simulink model "SkywalkerX8_Implementation"  (R2018a)
settings: Solver=FixedStepAuto  StartTime=0.0  StopTime=375  FixedStep=0.001  RelTol=1e-3
undefined symbols (not defined in the file): F, Light, MIL, SkywalkerX8
libraries: sensors x7, simulink_extras x3, aerolibwind2 x1
settings Model: Creator=David  LastModifiedBy=David

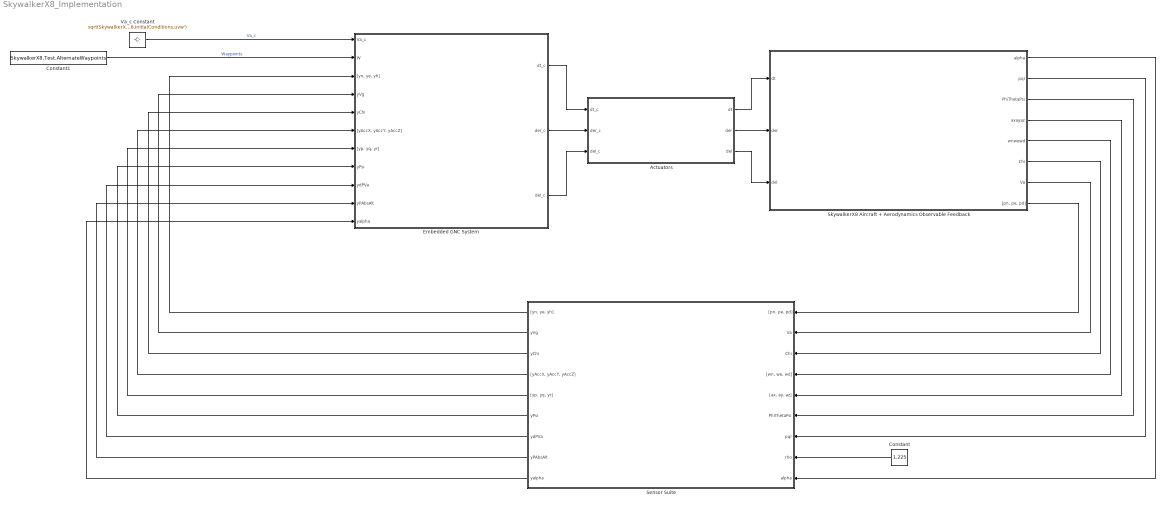
== system SkywalkerX8_Implementation ==
  Actuators : Subsystem
      mask Display:
      | image('actuators.jpg', 'center')
      | 
      | color('white')
      | 
      | port_label('input', 1, 'd_{t_c} (Unitless)', 'texmode', 'on')
      | port_label('input', 2, 'd_{{er}_c} (rad)', 'texmode', 'on')
      | port_label('input', 3, 'd_{{el}_c} (rad)', 'texmode', 'on')
      | 
      | port_label('output', 1, 'd_t (Unitless)', 'texmode', 'on')
      | port_label('output', 2, 'd_{er} (rad)', 'texmode', 'on')
      | port_label('output', 3, 'd_{el} (rad)', 'texmode', 'on')
  Constant : Constant  Value=1.225
  Constant1 : Constant  Value=SkywalkerX8.Test.AlternateWaypoints
  Embedded GNC System : Subsystem
      mask Display:
      | image('pixhawkv2-2.jpg')
      | 
      | color('cyan')
      | 
      | port_label('input', 1, 'Va_c (m/s)', 'texMode', 'On')
      | port_label('input', 2, '\bf{[W_i, W_{i+1} ..., W_N]} (m)', 'texMode', 'On')
      | port_label('input', 3, '[y_{GPS_N}, y_{GPS_E}, y_{GPS_h}] (m)', 'texMode', 'On')
      | port_label('input', 4, 'y_{GPS_{Vg}} (m/s)', 'texMode', 'On')
      | port_label('input', 5, 'y_{GPS_{\chi}} (rad)', 'texMode', 'On')
      | port_label('input', 6, '[y_{accel_x}, y_{accel_y}, y_{accel_z}] (m/s^2)', 'texMode', 'on')
      | port_label('input', 7, '[y_p, y_q, y_r] (rad/s)', 'texMode', 'on')
      | port_label('input', 8, 'y_{\psi} (rad)', 'texMode', 'on')
      | port_label('input', 9, 'y_{\DeltaP_{V_a}} (Pa)', 'texMode', 'on')
      | port_label('input', 10, 'y_{P_{abs}} (Pa)', 'texMode', 'on')
      | port_label('input', 11, 'y_\alpha (rad)', 'texMode', 'on')
      | 
      | port_label('output', 1, 'd_{t_c} (Unitless)', 'texmode', 'on')
      | port_label('output', 2, 'd_{{er}_c} (rad)', 'texmode', 'on')
      | port_label('output', 3, 'd_{{el}_c} (rad)', 'texmode', 'on')
  Sensor Suite : Subsystem
      mask Display:
      | image('telemetry.jpg')
      | 
      | color('cyan')
      | 
      | port_label('input', 1, '[p_N, p_E, p_D] (m)', 'texMode', 'On')
      | port_label('input', 2, 'V_a (m/s)', 'texMode', 'On')
      | port_label('input', 3, '\chi (rad)', 'texMode', 'On')
      | port_label('input', 4, '[w_N, w_E, w_D] (m/s)', 'texMode', 'On')
      | port_label('input', 5, '{\bfa_{inertial}} (m/s^2)', 'texMode', 'on')
      | port_label('input', 6, '[\phi, \theta, \psi] (rad)', 'texMode', 'on')
      | port_label('input', 7, '{\bf\omega_b} (rad/s)', 'texMode', 'on')
      | port_label('input', 8, '\rho (kg/m^3)', 'texMode', 'on')
      | port_label('input', 9, '\alpha (rad)', 'texMode', 'on')
      | 
      | port_label('output', 1, '[y_{GPS_N}, y_{GPS_E}, y_{GPS_h}] (m)', 'texMode', 'On')
      | port_label('output', 2, 'y_{GPS_{Vg}} (m/s)', 'texMode', 'On')
      | port_label('output', 3, 'y_{GPS_{\chi}} (rad)', 'texMode', 'On')
      | port_label('output', 4, '[y_{accel_x}, y_{accel_y}, y_{accel_z}] (m/s^2)', 'texMode', 'on')
      | port_label('output', 5, '[y_p, y_q, y_r] (rad/s)', 'texMode', 'on')
      | port_label('output', 6, 'y_{\psi} (rad)', 'texMode', 'on')
      | port_label('output', 7, 'y_{\DeltaP_{V_a}} (Pa)', 'texMode', 'on')
      | port_label('output', 8, 'y_{P_{abs}} (Pa)', 'texMode', 'on')
      | port_label('output', 9, 'y_\alpha (rad)', 'texMode', 'on')
  SkywalkerX8 Aircraft + Aerodynamics Observable Feedback : Subsystem
      mask Display:
      | image('x8SkySunset.png', 'center')
      | 
      | port_label('input', 1, '\delta_t (Unitless)', 'texmode', 'on')
      | port_label('input', 2, '\delta_e_r (rad)', 'texmode', 'on')
      | port_label('input', 3, '\delta_e_l (rad)', 'texmode', 'on')
      | 
      | port_label('output', 8, '[p_N, p_E, p_D] (m)', 'texMode', 'On')
      | port_label('output', 7, 'V_a (m/s)', 'texMode', 'On')
      | port_label('output', 6, '\chi (rad)', 'texMode', 'on')
      | port_label('output', 5, '[w_N, w_E, w_D] (m/s)', 'texMode', 'On')
      | port_label('output', 4, '{\bfa_{inertial}} (m/s^2)', 'texMode', 'on')
      | port_label('output', 3, '[\phi, \theta, \psi] (rad)', 'texMode', 'on')
      | port_label('output', 2, '{\bf\omega_b} (rad/s)', 'texMode', 'on')
      | port_label('output', 1, '\alpha (rad)', 'texMode', 'on')
  Va_c Constant : Constant  Value=sqrt(SkywalkerX8.InitialConditions.uvw*SkywalkerX8.InitialConditions.uvw')
  wires:
  SkywalkerX8 Aircraft + Aerodynamics Observable Feedback/3(PhiThetaPsi) -> Sensor Suite/6(PhiThetaPsi)
  SkywalkerX8 Aircraft + Aerodynamics Observable Feedback/8("[pn, pe, pd]") -> Sensor Suite/1("[pn, pe, pd]")
  SkywalkerX8 Aircraft + Aerodynamics Observable Feedback/6(Chi) -> Sensor Suite/3(Chi)
  SkywalkerX8 Aircraft + Aerodynamics Observable Feedback/2(pqr) -> Sensor Suite/7(pqr)
  Actuators/3(del) -> SkywalkerX8 Aircraft + Aerodynamics Observable Feedback/3(del)
  Constant/1 -> Sensor Suite/8(rho)
  SkywalkerX8 Aircraft + Aerodynamics Observable Feedback/4(axayaz) -> Sensor Suite/5("[ax, ay, az]")
  Actuators/1(dt) -> SkywalkerX8 Aircraft + Aerodynamics Observable Feedback/1(dt)
  SkywalkerX8 Aircraft + Aerodynamics Observable Feedback/5(wnwewd) -> Sensor Suite/4("[wn, we, wd]")
  SkywalkerX8 Aircraft + Aerodynamics Observable Feedback/7(Va) -> Sensor Suite/2(Va)
  SkywalkerX8 Aircraft + Aerodynamics Observable Feedback/1(alpha) -> Sensor Suite/9(alpha)
  Actuators/2(der) -> SkywalkerX8 Aircraft + Aerodynamics Observable Feedback/2(der)
  Va_c Constant/1 -> Embedded GNC System/1(Va_c)  "Va_c"
  Constant1/1 -> Embedded GNC System/2(W)  "Waypoints"
  Sensor Suite/1("[yn, ye, yh]") -> Embedded GNC System/3("[yn, ye, yh]")
  Sensor Suite/2(yVg) -> Embedded GNC System/4(yVg)
  Sensor Suite/3(yChi) -> Embedded GNC System/5(yChi)
  Sensor Suite/4("[yAccX, yAccY, yAccZ]") -> Embedded GNC System/6("[yAccX, yAccY, yAccZ]")
  Sensor Suite/5("[yp, yq, yr]") -> Embedded GNC System/7("[yp, yq, yr]")
  Sensor Suite/6(yPsi) -> Embedded GNC System/8(yPsi)
  Sensor Suite/7(ydPVa) -> Embedded GNC System/9(ydPVa)
  Sensor Suite/8(yPAbsAlt) -> Embedded GNC System/10(yPAbsAlt)
  Sensor Suite/9(yalpha) -> Embedded GNC System/11(yalpha)
  Embedded GNC System/1(dt_c) -> Actuators/1(dt_c)
  Embedded GNC System/2(der_c) -> Actuators/2(der_c)
  Embedded GNC System/3(del_c) -> Actuators/3(del_c)

== system SkywalkerX8_Implementation/Actuators ==
  dt_c : Inport
  der_c : Inport  Port=2
  del_c : Inport  Port=3
  Left Servo-Motor : Subsystem
      mask Display: image('servo.jpg', 'center')
  Motor Model : simulink_extras/Additional Linear/State-Space (with initial outputs)  A=SkywalkerX8.Actuators.Motor.SS.A  B=SkywalkerX8.Actuators.Motor.SS.B  C=SkywalkerX8.Actuators.Motor.SS.C  D=SkywalkerX8.Actuators.Motor.SS.D  U0=SkywalkerX8.InitialConditions.dt  Y0=SkywalkerX8.InitialConditions.dt  mask(State-Space with Initial Outputs){}
      settings: SourceProductName=Simulink  SourceProductBaseCode=SL
      mask Display: image('motor.jpg', 'center')
  Right Servo-Motor : Subsystem
      mask Display: image('servo.jpg', 'center')
  dt : Outport
  der : Outport  Port=2
  del : Outport  Port=3
  wires:
  del_c/1 -> Left Servo-Motor/1(del_c)
  Motor Model/1 -> dt/1
  Left Servo-Motor/1(del) -> del/1
  der_c/1 -> Right Servo-Motor/1(der_c)
  dt_c/1 -> Motor Model/1
  Right Servo-Motor/1(der) -> der/1

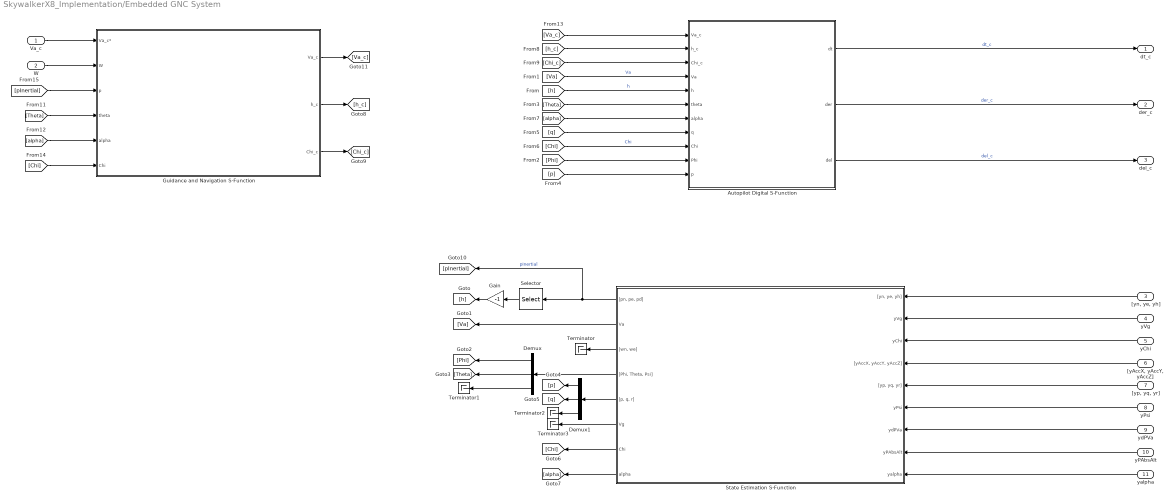
== system SkywalkerX8_Implementation/Embedded GNC System ==
  Va_c : Inport
  W : Inport  Port=2
  "[yn, ye, yh]" : Inport  Port=3
  yVg : Inport  Port=4
  yChi : Inport  Port=5
  "[yAccX, yAccY, yAccZ]" : Inport  Port=6
  "[yp, yq, yr]" : Inport  Port=7
  yPsi : Inport  Port=8
  ydPVa : Inport  Port=9
  yPAbsAlt : Inport  Port=10
  yalpha : Inport  Port=11
  Autopilot Digital S-Function : Subsystem
      mask help: Simulink:masks:GenSFuncDesc_MD
      mask Help: eval('feval(''rtwprivate'',''rtwhelpview'',''rtw_sfcn_block'')');
      mask Display:
      | image('autopilot.png', 'center')
      | 
      | port_label('output', 1, '\delta_t (Unitless)', 'texmode', 'on')
      | port_label('output', 2, '\delta_e_r (rad)', 'texmode', 'on')
      | port_label('output', 3, '\delta_e_l (rad)', 'texmode', 'on')
      | 
      | port_label('input', 1, 'V_{a_c} (m/s)', 'texmode', 'on')
      | port_label('input', 2, 'h_c (m)', 'texmode', 'on')
      | port_label('input', 3, '\chi_c (rad)', 'texmode', 'on')
      | port_label('input', 4, 'V_a (m/s)', 'texmode', 'on')
      | port_label('input', 5, 'Altitude (m)', 'texmode', 'on')
      | port_label('input', 6, '\theta (rad)', 'texmode', 'on')
      | port_label('input', 7, '\alpha (rad)', 'texmode', 'on')
      | port_label('input', 8, 'q (rad/s)', 'texmode', 'on')
      | port_label('input', 9, '\chi (rad)', 'texmode', 'on')
      | port_label('input', 10, '\phi (rad)', 'texmode', 'on')
      | port_label('input', 11, 'p (rad/s)', 'texmode', 'on')
  Demux : Demux  Outputs=3
  Demux1 : Demux  Outputs=3
  Gain : Gain  Gain=-1
  Guidance and Navigation S-Function : Subsystem
      mask help: Simulink:masks:GenSFuncDesc_MD
      mask Help: eval('feval(''rtwprivate'',''rtwhelpview'',''rtw_sfcn_block'')');
      mask Display:
      | image('Aircraft-navigation.jpg')
      | 
      | color('green')
      | 
      | port_label('input', 1, 'Va_c', 'texMode', 'On')
      | port_label('input', 2, '\bf{[W_1, W_2, ... W_n]}', 'texMode', 'On')
      | port_label('input', 3, '\bf{p}', 'texMode', 'On')
      | port_label('input', 4, '\theta', 'texMode', 'On')
      | port_label('input', 5, '\alpha', 'texMode', 'On')
      | port_label('input', 6, '\chi', 'texMode', 'On')
      | 
      | port_label('output', 1, 'Va_c', 'texMode', 'On')
      | port_label('output', 2, 'h_c', 'texMode', 'On')
      | port_label('output', 3, '\chi_c', 'texMode', 'On')
  Selector : Selector  InputPortWidth=3  IndexOptions=Index vector (dialog)  Indices=3  OutputSizes=1
  State Estimation S-Function : Subsystem
      mask help: Simulink:masks:GenSFuncDesc_MD
      mask Help: eval('feval(''rtwprivate'',''rtwhelpview'',''rtw_sfcn_block'')');
      mask Display:
      | image('state_estimate.jpg', 'center')
      | 
      | port_label('input', 1, '[y_{GPS_N}, y_{GPS_E}, y_{GPS_h}] (m)', 'texMode', 'On')
      | port_label('input', 2, 'y_{GPS_{Vg}} (m/s)', 'texMode', 'On')
      | port_label('input', 3, 'y_{GPS_{\chi}} (rad)', 'texMode', 'On')
      | port_label('input', 4, '[y_{accel_x}, y_{accel_y}, y_{accel_z}] (m/s^2)', 'texMode', 'on')
      | port_label('input', 5, '[y_p, y_q, y_r] (rad/s)', 'texMode', 'on')
      | port_label('input', 6, 'y_{\psi} (rad)', 'texMode', 'on')
      | port_label('input', 7, 'y_{\DeltaP_{V_a}} (Pa)', 'texMode', 'on')
      | port_label('input', 8, 'y_{P_{abs}} (Pa)', 'texMode', 'on')
      | port_label('input', 9, 'y_{\alpha} (rad)', 'texMode', 'on')
      | 
      | port_label('output', 1, '[p_N, p_E, p_D] (m)', 'texMode', 'On')
      | port_label('output', 2, 'V_a (m/s)', 'texMode', 'On')
      | port_label('output', 3, '[w_N, w_E] (m/s)', 'texMode', 'On')
      | port_label('output', 4, '[\phi, \theta, \psi] (rad)', 'texMode', 'on')
      | port_label('output', 5, '{\bf\omega_b} (rad/s)', 'texMode', 'on')
      | port_label('output', 6, 'V_g (m/s)', 'texMode', 'on')
      | port_label('output', 7, '\chi (rad)', 'texMode', 'on')
      | port_label('output', 8, '\alpha (rad)', 'texMode', 'on')
  Terminator{,1..3} (4 alike) : Terminator
  dt_c : Outport
  der_c : Outport  Port=2
  del_c : Outport  Port=3
  wires:
  [pInertial] -> Guidance and Navigation S-Function/3(p)
  "[yAccX, yAccY, yAccZ]"/1 -> State Estimation S-Function/4("[yAccX, yAccY, yAccZ]")
  State Estimation S-Function/6(Vg) -> Terminator3/1
  State Estimation S-Function/1("[pn, pe, pd]") -> [pInertial], Selector/1  "pInertial"
  [alpha] -> Autopilot Digital S-Function/7(alpha)
  Demux/2 -> [Theta]
  Demux1/3 -> Terminator2/1
  [h_c] -> Autopilot Digital S-Function/2(h_c)
  Demux/1 -> [Phi]
  Demux1/1 -> [p]
  [Chi] -> Guidance and Navigation S-Function/6(Chi)
  [q] -> Autopilot Digital S-Function/8(q)
  Demux/3 -> Terminator1/1
  [Phi] -> Autopilot Digital S-Function/10(Phi)
  yVg/1 -> State Estimation S-Function/2(yVg)
  W/1 -> Guidance and Navigation S-Function/2(W)
  Gain/1 -> [h]
  yPAbsAlt/1 -> State Estimation S-Function/8(yPAbsAlt)
  Selector/1 -> Gain/1
  Demux1/2 -> [q]
  [Chi_c] -> Autopilot Digital S-Function/3(Chi_c)
  "[yp, yq, yr]"/1 -> State Estimation S-Function/5("[yp, yq, yr]")
  yChi/1 -> State Estimation S-Function/3(yChi)
  [alpha] -> Guidance and Navigation S-Function/5(alpha)
  Guidance and Navigation S-Function/1(Va_c) -> [Va_c]
  Guidance and Navigation S-Function/3(Chi_c) -> [Chi_c]
  State Estimation S-Function/2(Va) -> [Va]
  State Estimation S-Function/7(Chi) -> [Chi]
  [Theta] -> Guidance and Navigation S-Function/4(theta)
  Guidance and Navigation S-Function/2(h_c) -> [h_c]
  State Estimation S-Function/4("[Phi, Theta, Psi]") -> Demux/1
  Autopilot Digital S-Function/1(dt) -> dt_c/1  "dt_c"
  State Estimation S-Function/3("[wn, we]") -> Terminator/1
  Autopilot Digital S-Function/2(der) -> der_c/1  "der_c"
  State Estimation S-Function/8(alpha) -> [alpha]
  Va_c/1 -> Guidance and Navigation S-Function/1(Va_c*)
  Autopilot Digital S-Function/3(del) -> del_c/1  "del_c"
  State Estimation S-Function/5("[p, q, r]") -> Demux1/1
  "[yn, ye, yh]"/1 -> State Estimation S-Function/1("[yn, ye, yh]")
  [Theta] -> Autopilot Digital S-Function/6(theta)
  [Va_c] -> Autopilot Digital S-Function/1(Va_c)
  yPsi/1 -> State Estimation S-Function/6(yPsi)
  [Va] -> Autopilot Digital S-Function/4(Va)  "Va"
  [p] -> Autopilot Digital S-Function/11(p)
  [h] -> Autopilot Digital S-Function/5(h)  "h"
  [Chi] -> Autopilot Digital S-Function/9(Chi)  "Chi"
  yalpha/1 -> State Estimation S-Function/9(yalpha)
  ydPVa/1 -> State Estimation S-Function/7(ydPVa)

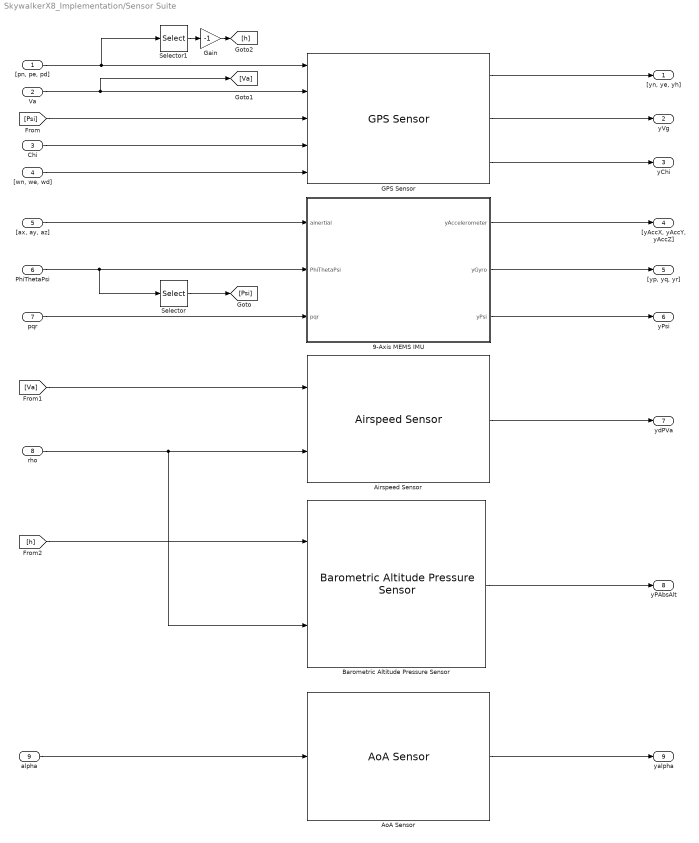
== system SkywalkerX8_Implementation/Sensor Suite ==
  "[pn, pe, pd]" : Inport
  Va : Inport  Port=2
  Chi : Inport  Port=3
  "[wn, we, wd]" : Inport  Port=4
  "[ax, ay, az]" : Inport  Port=5
  PhiThetaPsi : Inport  Port=6
  pqr : Inport  Port=7
  rho : Inport  Port=8
  alpha : Inport  Port=9
  9-Axis MEMS IMU : Subsystem
      mask Display:
      | image('VNAV_IMU.jpg')
      | 
      | color('green')
      | 
      | port_label('input', 1, '{\bfa_{inertial}} (m/s^2)', 'texMode', 'on')
      | port_label('input', 2, '[\phi, \theta, \psi] (rad)', 'texMode', 'on')
      | port_label('input', 3, '{\bf\omega_b} (rad/s)', 'texMode', 'on')
      | 
      | port_label('output', 1, '[y_{accel_x}, y_{accel_y}, y_{accel_z}] (m/s^2)', 'texMode', 'on')
      | port_label('output', 2, '[y_p, y_q, y_r] (rad/s)', 'texMode', 'on')
      | port_label('output', 3, 'y_{\psi} (rad)', 'texMode', 'on')
  Airspeed Sensor : sensors/Airspeed Sensor  SampleTime=SkywalkerX8.Sensors.AirspeedPressure.SampleTime  diffPressureStdDev=SkywalkerX8.Sensors.AirspeedPressure.StdDev  diffPressureBandwidthHz=SkywalkerX8.Sensors.AirspeedPressure.BandwidthHz  diffPressureInit=SkywalkerX8.Sensors.AirspeedPressure.InitialCondition  diffPressureUpperSaturation=SkywalkerX8.Sensors.AirspeedPressure.UpperSat  diffPressureLowerSaturation=SkywalkerX8.Sensors.AirspeedPressure.LowerSat  diffPressureResolution=SkywalkerX8.Sensors.AirspeedPressure.Resolution
  AoA Sensor : sensors/AoA Sensor  SampleTime=SkywalkerX8.Sensors.AoA.SampleTime  alphaStdDev=SkywalkerX8.Sensors.AoA.StdDev  alphaBandwidthHz=SkywalkerX8.Sensors.AoA.BandwidthHz  alphaInit=SkywalkerX8.Sensors.AoA.InitialCondition  alphaUpperSaturation=SkywalkerX8.Sensors.AoA.UpperSat  alphaLowerSaturation=SkywalkerX8.Sensors.AoA.LowerSat  alphaResolution=SkywalkerX8.Sensors.AoA.Resolution
  Barometric Altitude Pressure Sensor : sensors/Barometric Altitude Pressure Sensor  g=SkywalkerX8.System.Gravity  SampleTime=SkywalkerX8.Sensors.AltitudePressure.SampleTime  absPressureStdDev=SkywalkerX8.Sensors.AltitudePressure.StdDev  absPressureBandwidthHz=SkywalkerX8.Sensors.AltitudePressure.BandwidthHz  absPressureInit=SkywalkerX8.Sensors.AltitudePressure.InitialCondition  absPressureUpperSaturation=SkywalkerX8.Sensors.AltitudePressure.UpperSat  absPressureLowerSaturation=SkywalkerX8.Sensors.AltitudePressure.LowerSat  absPressureResolution=SkywalkerX8.Sensors.AltitudePressure.Resolution
  GPS Sensor : sensors/GPS Sensor  SampleTime=SkywalkerX8.Sensors.GPS.SampleTime  pnInit=SkywalkerX8.Sensors.GPS.pnInit  peInit=SkywalkerX8.Sensors.GPS.peInit  pdInit=SkywalkerX8.Sensors.GPS.pdInit  VgInit=SkywalkerX8.Sensors.GPS.VgInit  ChiInit=SkywalkerX8.Sensors.GPS.ChiInit  GPSNStdDev=SkywalkerX8.Sensors.GPS.North.StdDev  OneOverkGPSN=SkywalkerX8.Sensors.GPS.North.TimeConstant  GPSEStdDev=SkywalkerX8.Sensors.GPS.East.StdDev  OneOverkGPSE=SkywalkerX8.Sensors.GPS.East.TimeConstant  GPSAltStdDev=SkywalkerX8.Sensors.GPS.Alt.StdDev  OneOverkGPSAlt=SkywalkerX8.Sensors.GPS.Alt.TimeConstant  GPSVStdDev=SkywalkerX8.Sensors.GPS.Velocity.StdDev
  Gain : Gain  Gain=-1
  Selector : Selector  InputPortWidth=3  IndexOptions=Index vector (dialog)  Indices=3  OutputSizes=1
  Selector1 : Selector  InputPortWidth=3  IndexOptions=Index vector (dialog)  Indices=3  OutputSizes=1
  "[yn, ye, yh]" : Outport
  yVg : Outport  Port=2
  yChi : Outport  Port=3
  "[yAccX, yAccY, yAccZ]" : Outport  Port=4
  "[yp, yq, yr]" : Outport  Port=5
  yPsi : Outport  Port=6
  ydPVa : Outport  Port=7
  yPAbsAlt : Outport  Port=8
  yalpha : Outport  Port=9
  wires:
  "[pn, pe, pd]"/1 -> GPS Sensor/1, Selector1/1
  Va/1 -> [Va], GPS Sensor/2
  PhiThetaPsi/1 -> 9-Axis MEMS IMU/2(PhiThetaPsi), Selector/1
  Airspeed Sensor/1 -> ydPVa/1
  [Psi] -> GPS Sensor/3
  Selector1/1 -> Gain/1
  rho/1 -> Barometric Altitude Pressure Sensor/2, Airspeed Sensor/2
  GPS Sensor/3 -> yChi/1
  Selector/1 -> [Psi]
  [h] -> Barometric Altitude Pressure Sensor/1
  9-Axis MEMS IMU/3(yPsi) -> yPsi/1
  [Va] -> Airspeed Sensor/1
  pqr/1 -> 9-Axis MEMS IMU/3(pqr)
  9-Axis MEMS IMU/2(yGyro) -> "[yp, yq, yr]"/1
  "[wn, we, wd]"/1 -> GPS Sensor/5
  Barometric Altitude Pressure Sensor/1 -> yPAbsAlt/1
  GPS Sensor/1 -> "[yn, ye, yh]"/1
  Gain/1 -> [h]
  GPS Sensor/2 -> yVg/1
  "[ax, ay, az]"/1 -> 9-Axis MEMS IMU/1(ainertial)
  9-Axis MEMS IMU/1(yAccelerometer) -> "[yAccX, yAccY, yAccZ]"/1
  AoA Sensor/1 -> yalpha/1
  alpha/1 -> AoA Sensor/1
  Chi/1 -> GPS Sensor/4

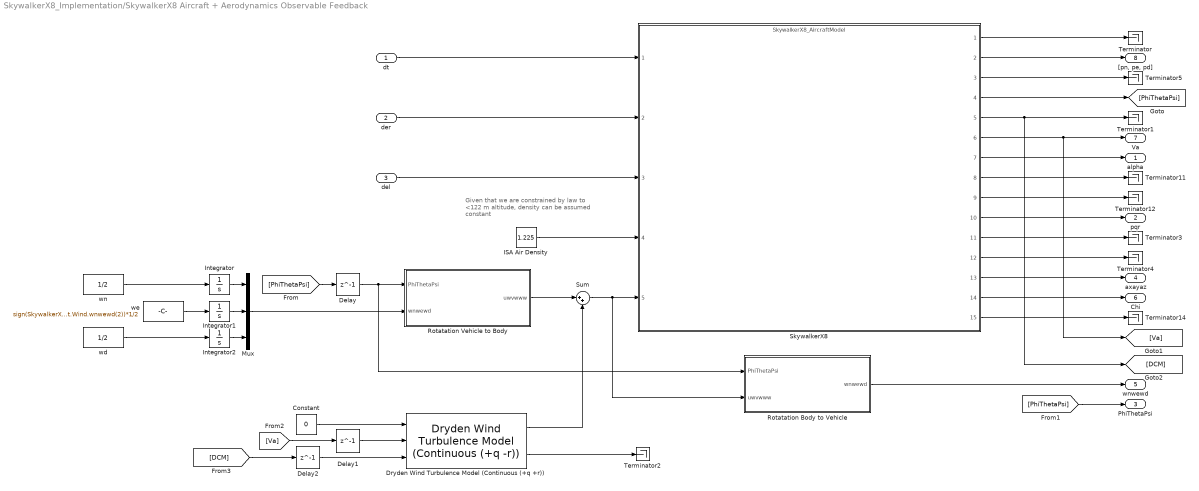
== system SkywalkerX8_Implementation/SkywalkerX8 Aircraft + Aerodynamics Observable Feedback ==
  note: Given that we are constrained by law to
      | <122 m altitude, density can be assumed
      | constant
  dt : Inport
  der : Inport  Port=2
  del : Inport  Port=3
  Constant : Constant  Value=0
  Delay : Delay  DelayLength=1  InitialCondition=SkywalkerX8.InitialConditions.PhiThetaPsi
  Delay1 : Delay  DelayLength=1  InitialCondition=sqrt(SkywalkerX8.InitialConditions.uvw*SkywalkerX8.InitialConditions.uvw')
  Delay2 : Delay  DelayLength=1  InitialCondition=zeros(3, 3)
  Dryden Wind Turbulence Model (Continuous (+q +r)) : aerolibwind2/Dryden Wind Turbulence Model  (Continuous (+q -r))  units=Metric (MKS)  spec=MIL-F-8785C  model=Continuous Dryden (+q +r)  W20=sqrt(SkywalkerX8.Ambient.Wind.wnwewd*SkywalkerX8.Ambient.Wind.wnwewd')  Wdeg=rad2deg(atan2(SkywalkerX8.Ambient.Wind.wnwewd(2), SkywalkerX8.Ambient.Wind.wnwewd(1)))  TurbProb=10^-2 - Light  L_high=533.4  Wingspan=SkywalkerX8.Geometry.b  ts=0.001  Seed=[23341 23342 23343 23344]  T_on=on
      settings: SourceProductName=Aerospace Blockset
  ISA Air Density : Constant  Value=1.225
  Integrator : Integrator  LimitOutput=on  UpperSaturationLimit=(SkywalkerX8.Ambient.Wind.wnwewd(1)>0)*SkywalkerX8.Ambient.Wind.wnwewd(1)+1E-06  LowerSaturationLimit=(SkywalkerX8.Ambient.Wind.wnwewd(1)<0)*SkywalkerX8.Ambient.Wind.wnwewd(1)-1E-06
  Integrator1 : Integrator  LimitOutput=on  UpperSaturationLimit=(SkywalkerX8.Ambient.Wind.wnwewd(2)>0)*SkywalkerX8.Ambient.Wind.wnwewd(2)+1E-06  LowerSaturationLimit=(SkywalkerX8.Ambient.Wind.wnwewd(2)<0)*SkywalkerX8.Ambient.Wind.wnwewd(2)-1E-06
  Integrator2 : Integrator  LimitOutput=on  UpperSaturationLimit=(SkywalkerX8.Ambient.Wind.wnwewd(3)>0)*SkywalkerX8.Ambient.Wind.wnwewd(3)+1E-06  LowerSaturationLimit=(SkywalkerX8.Ambient.Wind.wnwewd(3)<0)*SkywalkerX8.Ambient.Wind.wnwewd(3)-1E-06
  Mux : Mux  Inputs=3
  Rotatation Body to Vehicle : MATLAB Function  TreatAsAtomicUnit=on
  Rotatation Vehicle to Body : MATLAB Function  TreatAsAtomicUnit=on
  SkywalkerX8 : ModelReference  ModelNameDialog=SkywalkerX8_AircraftModel  ModelReferenceVersion=1.367
      mask Display:
      | image('C:\MATLAB\masters\icons\Skywalker Main Block Icon.png', 'center')
      | 
      | color('cyan')
      | 
      | port_label('input', 1, 'k_{motor} (Unitless)', 'texmode', 'on')
      | port_label('input', 2, '\delta_{er} (rad)', 'texmode', 'on')
      | port_label('input', 3, '\delta_{el} (rad)', 'texmode', 'on')
      | port_label('input', 4, '\rho (kg/m^3)', 'texmode', 'on')
      | port_label('input', 5, '{\bf V_w^b} (m/s)', 'texmode', 'on')
      | 
      | port_label('output', 1, '{\bf V_e} (m/s)', 'texmode', 'on')
      | port_label('output', 2, '{\bf X_e} (m)', 'texmode', 'on')
      | port_label('output', 3, 'Altitude (m)', 'texmode', 'on')
      | port_label('output', 4, '\phi \theta \psi (rad)', 'texmode', 'on')
      | port_label('output', 5, 'R_{inertial}^{body}', 'texmode', 'on')
      | port_label('output', 6, 'V_a (m/s)', 'texmode', 'on')
      | port_label('output', 7, 'alpha (rad)', 'texmode', 'on')
      | port_label('output', 8, 'beta (rad)', 'texmode', 'on')
      | port_label('output', 9, '{\bf V_b} (m/s)', 'texmode', 'on')
      | port_label('output', 10, '{\bf \omega_b} (rad/s)', 'texmode', 'on')
      | port_label('output', 11, '{\bf \delta\omega_b/\deltat} (rad/s^2)', 'texmode', 'on')
      | port_label('output', 12, '{\bf a_{body}} (m/s^2)', 'texmode', 'on')
      | port_label('output', 13, '{\bf a_{inertial}} (m/s^2)', 'texmode', 'on')
      | port_label('output', 14, '\chi (rad)', 'texmode', 'on')
      | port_label('output', 15, '\chi_c (rad)', 'texmode', 'on')
  Sum : Sum  Inputs=|++
  Terminator{,1..5,11..12,14} (9 alike) : Terminator
  wd : Constant  Value=1/2
  we : Constant  Value=sign(SkywalkerX8.Ambient.Wind.wnwewd(2))*1/2
  wn : Constant  Value=1/2
  alpha : Outport
  pqr : Outport  Port=2
  PhiThetaPsi : Outport  Port=3
  axayaz : Outport  Port=4
  wnwewd : Outport  Port=5
  Chi : Outport  Port=6
  Va : Outport  Port=7
  "[pn, pe, pd]" : Outport  Port=8
  wires:
  SkywalkerX8/12 -> Terminator4/1
  SkywalkerX8/13 -> axayaz/1
  Rotatation Vehicle to Body/1(uwvwww) -> Sum/1
  SkywalkerX8/11 -> Terminator3/1
  SkywalkerX8/6 -> [Va], Va/1
  SkywalkerX8/1 -> Terminator/1
  SkywalkerX8/5 -> [DCM], Terminator1/1
  SkywalkerX8/7 -> alpha/1
  dt/1 -> SkywalkerX8/1
  SkywalkerX8/8 -> Terminator11/1
  SkywalkerX8/3 -> Terminator5/1
  SkywalkerX8/9 -> Terminator12/1
  SkywalkerX8/2 -> "[pn, pe, pd]"/1
  SkywalkerX8/4 -> [PhiThetaPsi]
  SkywalkerX8/15 -> Terminator14/1
  SkywalkerX8/10 -> pqr/1
  ISA Air Density/1 -> SkywalkerX8/4
  SkywalkerX8/14 -> Chi/1
  del/1 -> SkywalkerX8/3
  der/1 -> SkywalkerX8/2
  Mux/1 -> Rotatation Vehicle to Body/2(wnwewd)
  [PhiThetaPsi] -> Delay/1
  [PhiThetaPsi] -> PhiThetaPsi/1
  Delay/1 -> Rotatation Body to Vehicle/1(PhiThetaPsi), Rotatation Vehicle to Body/1(PhiThetaPsi)
  Constant/1 -> Dryden Wind Turbulence Model (Continuous (+q +r))/1
  [Va] -> Delay1/1
  [DCM] -> Delay2/1
  Dryden Wind Turbulence Model (Continuous (+q +r))/2 -> Terminator2/1
  Sum/1 -> Rotatation Body to Vehicle/2(uwvwww), SkywalkerX8/5
  Dryden Wind Turbulence Model (Continuous (+q +r))/1 -> Sum/2
  Delay1/1 -> Dryden Wind Turbulence Model (Continuous (+q +r))/2
  Delay2/1 -> Dryden Wind Turbulence Model (Continuous (+q +r))/3
  Rotatation Body to Vehicle/1(wnwewd) -> wnwewd/1
  wd/1 -> Integrator2/1
  Integrator2/1 -> Mux/3
  wn/1 -> Integrator/1
  Integrator/1 -> Mux/1
  we/1 -> Integrator1/1
  Integrator1/1 -> Mux/2

== system SkywalkerX8_Implementation/Actuators/Left Servo-Motor ==
  del_c : Inport
  Rate Limiter : RateLimiter  Commented=through  RisingSlewLimit=SkywalkerX8.Actuators.Servos.RateLimit  FallingSlewLimit=-SkywalkerX8.Actuators.Servos.RateLimit  SampleTimeMode=inherited  InitialCondition=SkywalkerX8.InitialConditions.de*0.5 + SkywalkerX8.InitialConditions.da*0.5
  Saturation : Saturate  UpperLimit=SkywalkerX8.Actuators.Servos.UpperSaturation  LowerLimit=SkywalkerX8.Actuators.Servos.LowerSaturation
  Second Order Servo-Motor Model : simulink_extras/Additional Linear/State-Space (with initial outputs)  A=SkywalkerX8.Actuators.Servos.SS.A  B=SkywalkerX8.Actuators.Servos.SS.B  C=SkywalkerX8.Actuators.Servos.SS.C  D=SkywalkerX8.Actuators.Servos.SS.D  U0=(SkywalkerX8.InitialConditions.de*0.5 + SkywalkerX8.InitialConditions.da*0.5)  Y0=(SkywalkerX8.InitialConditions.de*0.5 + SkywalkerX8.InitialConditions.da*0.5)
      settings: SourceProductName=Simulink  SourceProductBaseCode=SL
  del : Outport
  wires:
  Rate Limiter/1 -> Saturation/1
  del_c/1 -> Second Order Servo-Motor Model/1
  Saturation/1 -> del/1
  Second Order Servo-Motor Model/1 -> Rate Limiter/1

== system SkywalkerX8_Implementation/Actuators/Right Servo-Motor ==
  der_c : Inport
  Rate Limiter : RateLimiter  Commented=through  RisingSlewLimit=SkywalkerX8.Actuators.Servos.RateLimit  FallingSlewLimit=-SkywalkerX8.Actuators.Servos.RateLimit  SampleTimeMode=inherited  InitialCondition=SkywalkerX8.InitialConditions.de*0.5 - SkywalkerX8.InitialConditions.da*0.5
  Saturation : Saturate  UpperLimit=SkywalkerX8.Actuators.Servos.UpperSaturation  LowerLimit=SkywalkerX8.Actuators.Servos.LowerSaturation
  Second Order Servo-Motor Model : simulink_extras/Additional Linear/State-Space (with initial outputs)  A=SkywalkerX8.Actuators.Servos.SS.A  B=SkywalkerX8.Actuators.Servos.SS.B  C=SkywalkerX8.Actuators.Servos.SS.C  D=SkywalkerX8.Actuators.Servos.SS.D  U0=(SkywalkerX8.InitialConditions.de*0.5 - SkywalkerX8.InitialConditions.da*0.5)  Y0=(SkywalkerX8.InitialConditions.de*0.5 - SkywalkerX8.InitialConditions.da*0.5)
      settings: SourceProductName=Simulink  SourceProductBaseCode=SL
  der : Outport
  wires:
  Rate Limiter/1 -> Saturation/1
  der_c/1 -> Second Order Servo-Motor Model/1
  Second Order Servo-Motor Model/1 -> Rate Limiter/1
  Saturation/1 -> der/1

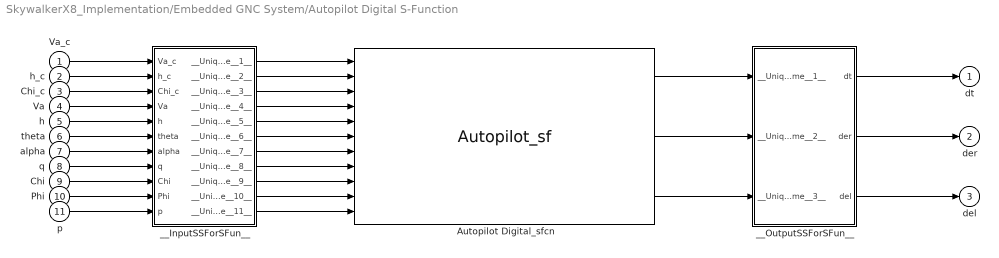
== system SkywalkerX8_Implementation/Embedded GNC System/Autopilot Digital S-Function ==
  Va_c : Inport
  h_c : Inport  Port=2
  Chi_c : Inport  Port=3
  Va : Inport  Port=4
  h : Inport  Port=5
  theta : Inport  Port=6
  alpha : Inport  Port=7
  q : Inport  Port=8
  Chi : Inport  Port=9
  Phi : Inport  Port=10
  p : Inport  Port=11
  Autopilot Digital_sfcn : S-Function  FunctionName=Autopilot_sf  SFunctionModules=""  SFunctionDeploymentMode=off  EnableBusSupport=off  SFcnStateName=DWORK0  mask{rtw_sf_name=Autopilot_sf, showVar=off}
      mask prompts: rtw_sf_name "Simulink:masks:GenSFuncName_MP"; showVar "Simulink:masks:GenSFuncShowModuleList_MP"
      mask help: Simulink:masks:GenSFuncDesc_MD
      mask init:
      | displist = '';
      | if ~strcmp(get_param(gcb, 'FunctionName'), rtw_sf_name);
      |   set_param(gcb, 'FunctionName', rtw_sf_name);
      | end
      | % Check if we are generating code
      | rtw_mode = false;
      | if strcmpi(get_param(bdroot(gcb),'SimulationStatus'),'Initializing')
      | 	rtw_mode = strcmpi(get_param(bdroot(gcb),'BuildingRTWCode'),'on') && ...
      | 		~strcmpi(get_param(bdroot(gcb),'TargetStyle'),'SimulationTarget');
      | end
      | if showVar || rtw_mode
      | 	if exist('rtwsfunc') == 2 | exist('rtwsfunc') == 6
      | 		tmplist = rtwsfunc(rtw_sf_name,gcb);
      | 		tmplist = DAStudio.message('Simulink:masks:GenSFuncListOfModules_IC', tmplist);
      | 	elseif showVar
      | 		tmplist1 = DAStudio.message('Simulink:masks:GenSFuncListOfModules_IC', '');
      |         tmplist2 = DAStudio.message('Simulink:masks:GenSFuncNotLicensed_IC');
      |         tmplist = [tmplist1 tmplist2];
      |  	end
      | end
      | if showVar
      |   displist = tmplist;
      | end
      settings: SFcnIsStateOwnerBlock=on
      settings: CopyFcn=|
      | if ~strcmp(get_param(gcb,'Linkstatus'),'none') && ...
      | ~strcmp(get_param(gcb,'Linkstatus'),'implicit')
      |   set_param(gcb,'LinkStatus','none');
      | end
      mask Help: eval('feval(''rtwprivate'',''rtwhelpview'',''rtw_sfcn_block'')');
      mask Display:
      | port_label('input',1,'Va_c');
      | port_label('input',2,'h_c');
      | port_label('input',3,'Chi_c');
      | port_label('input',4,'Va');
      | port_label('input',5,'h');
      | port_label('input',6,'theta');
      | port_label('input',7,'alpha');
      | port_label('input',8,'q');
      | port_label('input',9,'Chi');
      | port_label('input',10,'Phi');
      | port_label('input',11,'p');
      | port_label('output',1,'dt');
      | port_label('output',2,'der');
      | port_label('output',3,'del');
  __InputSSForSFun__ : Subsystem
  __OutputSSForSFun__ : Subsystem
  dt : Outport
  der : Outport  Port=2
  del : Outport  Port=3
  wires:
  Va_c/1 -> __InputSSForSFun__/1(Va_c)
  h_c/1 -> __InputSSForSFun__/2(h_c)
  Chi_c/1 -> __InputSSForSFun__/3(Chi_c)
  Va/1 -> __InputSSForSFun__/4(Va)
  h/1 -> __InputSSForSFun__/5(h)
  theta/1 -> __InputSSForSFun__/6(theta)
  alpha/1 -> __InputSSForSFun__/7(alpha)
  q/1 -> __InputSSForSFun__/8(q)
  Chi/1 -> __InputSSForSFun__/9(Chi)
  Phi/1 -> __InputSSForSFun__/10(Phi)
  p/1 -> __InputSSForSFun__/11(p)
  __InputSSForSFun__/1(__UniqueOutportName__1__) -> Autopilot Digital_sfcn/1
  __InputSSForSFun__/2(__UniqueOutportName__2__) -> Autopilot Digital_sfcn/2
  __InputSSForSFun__/3(__UniqueOutportName__3__) -> Autopilot Digital_sfcn/3
  __InputSSForSFun__/4(__UniqueOutportName__4__) -> Autopilot Digital_sfcn/4
  __InputSSForSFun__/5(__UniqueOutportName__5__) -> Autopilot Digital_sfcn/5
  __InputSSForSFun__/6(__UniqueOutportName__6__) -> Autopilot Digital_sfcn/6
  __InputSSForSFun__/7(__UniqueOutportName__7__) -> Autopilot Digital_sfcn/7
  __InputSSForSFun__/8(__UniqueOutportName__8__) -> Autopilot Digital_sfcn/8
  __InputSSForSFun__/9(__UniqueOutportName__9__) -> Autopilot Digital_sfcn/9
  __InputSSForSFun__/10(__UniqueOutportName__10__) -> Autopilot Digital_sfcn/10
  __InputSSForSFun__/11(__UniqueOutportName__11__) -> Autopilot Digital_sfcn/11
  Autopilot Digital_sfcn/1 -> __OutputSSForSFun__/1(__UniqueInportName__1__)
  Autopilot Digital_sfcn/2 -> __OutputSSForSFun__/2(__UniqueInportName__2__)
  Autopilot Digital_sfcn/3 -> __OutputSSForSFun__/3(__UniqueInportName__3__)
  __OutputSSForSFun__/1(dt) -> dt/1
  __OutputSSForSFun__/2(der) -> der/1
  __OutputSSForSFun__/3(del) -> del/1

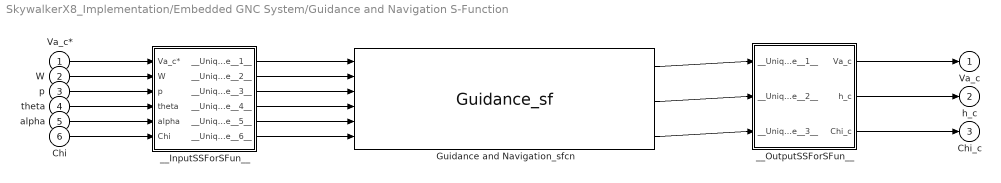
== system SkywalkerX8_Implementation/Embedded GNC System/Guidance and Navigation S-Function ==
  Va_c* : Inport
  W : Inport  Port=2
  p : Inport  Port=3
  theta : Inport  Port=4
  alpha : Inport  Port=5
  Chi : Inport  Port=6
  Guidance and Navigation_sfcn : S-Function  FunctionName=Guidance_sf  SFunctionModules=""  SFunctionDeploymentMode=off  EnableBusSupport=off  SFcnStateName=DWORK0  mask{rtw_sf_name=Guidance_sf, showVar=off}
      mask prompts: rtw_sf_name "Simulink:masks:GenSFuncName_MP"; showVar "Simulink:masks:GenSFuncShowModuleList_MP"
      mask help: Simulink:masks:GenSFuncDesc_MD
      mask init: same as SkywalkerX8_Implementation/Embedded GNC System/Autopilot Digital S-Function/Autopilot Digital_sfcn
      settings: SFcnIsStateOwnerBlock=on
      settings: CopyFcn=|
      | if ~strcmp(get_param(gcb,'Linkstatus'),'none') && ...
      | ~strcmp(get_param(gcb,'Linkstatus'),'implicit')
      |   set_param(gcb,'LinkStatus','none');
      | end
      mask Help: eval('feval(''rtwprivate'',''rtwhelpview'',''rtw_sfcn_block'')');
      mask Display:
      | port_label('input',1,'Va_c*');
      | port_label('input',2,'W');
      | port_label('input',3,'p');
      | port_label('input',4,'theta');
      | port_label('input',5,'alpha');
      | port_label('input',6,'Chi');
      | port_label('output',1,'Va_c');
      | port_label('output',2,'h_c');
      | port_label('output',3,'Chi_c');
  __InputSSForSFun__ : Subsystem
  __OutputSSForSFun__ : Subsystem
  Va_c : Outport
  h_c : Outport  Port=2
  Chi_c : Outport  Port=3
  wires:
  Va_c*/1 -> __InputSSForSFun__/1(Va_c*)
  W/1 -> __InputSSForSFun__/2(W)
  p/1 -> __InputSSForSFun__/3(p)
  theta/1 -> __InputSSForSFun__/4(theta)
  alpha/1 -> __InputSSForSFun__/5(alpha)
  Chi/1 -> __InputSSForSFun__/6(Chi)
  __InputSSForSFun__/1(__UniqueOutportName__1__) -> Guidance and Navigation_sfcn/1
  __InputSSForSFun__/2(__UniqueOutportName__2__) -> Guidance and Navigation_sfcn/2
  __InputSSForSFun__/3(__UniqueOutportName__3__) -> Guidance and Navigation_sfcn/3
  __InputSSForSFun__/4(__UniqueOutportName__4__) -> Guidance and Navigation_sfcn/4
  __InputSSForSFun__/5(__UniqueOutportName__5__) -> Guidance and Navigation_sfcn/5
  __InputSSForSFun__/6(__UniqueOutportName__6__) -> Guidance and Navigation_sfcn/6
  Guidance and Navigation_sfcn/1 -> __OutputSSForSFun__/1(__UniqueInportName__1__)
  Guidance and Navigation_sfcn/2 -> __OutputSSForSFun__/2(__UniqueInportName__2__)
  Guidance and Navigation_sfcn/3 -> __OutputSSForSFun__/3(__UniqueInportName__3__)
  __OutputSSForSFun__/1(Va_c) -> Va_c/1
  __OutputSSForSFun__/2(h_c) -> h_c/1
  __OutputSSForSFun__/3(Chi_c) -> Chi_c/1

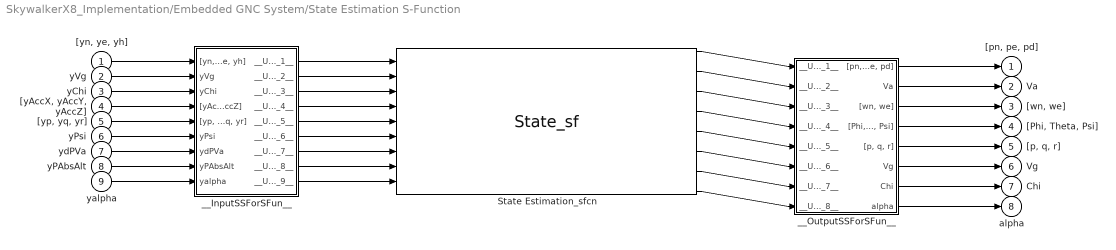
== system SkywalkerX8_Implementation/Embedded GNC System/State Estimation S-Function ==
  "[yn, ye, yh]" : Inport  PortDimensions=3
  yVg : Inport  Port=2
  yChi : Inport  Port=3
  "[yAccX, yAccY, yAccZ]" : Inport  Port=4  PortDimensions=3
  "[yp, yq, yr]" : Inport  Port=5  PortDimensions=3
  yPsi : Inport  Port=6
  ydPVa : Inport  Port=7
  yPAbsAlt : Inport  Port=8
  yalpha : Inport  Port=9
  State Estimation_sfcn : S-Function  FunctionName=State_sf  SFunctionModules=""  SFunctionDeploymentMode=off  EnableBusSupport=off  SFcnStateName=DWORK0  mask{rtw_sf_name=State_sf, showVar=off}
      mask prompts: rtw_sf_name "Simulink:masks:GenSFuncName_MP"; showVar "Simulink:masks:GenSFuncShowModuleList_MP"
      mask help: Simulink:masks:GenSFuncDesc_MD
      mask init: same as SkywalkerX8_Implementation/Embedded GNC System/Autopilot Digital S-Function/Autopilot Digital_sfcn
      settings: SFcnIsStateOwnerBlock=on
      settings: CopyFcn=|
      | if ~strcmp(get_param(gcb,'Linkstatus'),'none') && ...
      | ~strcmp(get_param(gcb,'Linkstatus'),'implicit')
      |   set_param(gcb,'LinkStatus','none');
      | end
      mask Help: eval('feval(''rtwprivate'',''rtwhelpview'',''rtw_sfcn_block'')');
      mask Display:
      | port_label('input',1,'[yn, ye, yh]');
      | port_label('input',2,'yVg');
      | port_label('input',3,'yChi');
      | port_label('input',4,'[yAccX, yAccY, yAccZ]');
      | port_label('input',5,'[yp, yq, yr]');
      | port_label('input',6,'yPsi');
      | port_label('input',7,'ydPVa');
      | port_label('input',8,'yPAbsAlt');
      | port_label('input',9,'yalpha');
      | port_label('output',1,'[pn, pe, pd]');
      | port_label('output',2,'Va');
      | port_label('output',3,'[wn, we]');
      | port_label('output',4,'[Phi, Theta, Psi]');
      | port_label('output',5,'[p, q, r]');
      | port_label('output',6,'Vg');
      | port_label('output',7,'Chi');
      | port_label('output',8,'alpha');
  __InputSSForSFun__ : Subsystem
  __OutputSSForSFun__ : Subsystem
  "[pn, pe, pd]" : Outport
  Va : Outport  Port=2
  "[wn, we]" : Outport  Port=3
  "[Phi, Theta, Psi]" : Outport  Port=4
  "[p, q, r]" : Outport  Port=5
  Vg : Outport  Port=6
  Chi : Outport  Port=7
  alpha : Outport  Port=8
  wires:
  "[yn, ye, yh]"/1 -> __InputSSForSFun__/1("[yn, ye, yh]")
  yVg/1 -> __InputSSForSFun__/2(yVg)
  yChi/1 -> __InputSSForSFun__/3(yChi)
  "[yAccX, yAccY, yAccZ]"/1 -> __InputSSForSFun__/4("[yAccX, yAccY, yAccZ]")
  "[yp, yq, yr]"/1 -> __InputSSForSFun__/5("[yp, yq, yr]")
  yPsi/1 -> __InputSSForSFun__/6(yPsi)
  ydPVa/1 -> __InputSSForSFun__/7(ydPVa)
  yPAbsAlt/1 -> __InputSSForSFun__/8(yPAbsAlt)
  yalpha/1 -> __InputSSForSFun__/9(yalpha)
  __InputSSForSFun__/1(__UniqueOutportName__1__) -> State Estimation_sfcn/1
  __InputSSForSFun__/2(__UniqueOutportName__2__) -> State Estimation_sfcn/2
  __InputSSForSFun__/3(__UniqueOutportName__3__) -> State Estimation_sfcn/3
  __InputSSForSFun__/4(__UniqueOutportName__4__) -> State Estimation_sfcn/4
  __InputSSForSFun__/5(__UniqueOutportName__5__) -> State Estimation_sfcn/5
  __InputSSForSFun__/6(__UniqueOutportName__6__) -> State Estimation_sfcn/6
  __InputSSForSFun__/7(__UniqueOutportName__7__) -> State Estimation_sfcn/7
  __InputSSForSFun__/8(__UniqueOutportName__8__) -> State Estimation_sfcn/8
  __InputSSForSFun__/9(__UniqueOutportName__9__) -> State Estimation_sfcn/9
  State Estimation_sfcn/1 -> __OutputSSForSFun__/1(__UniqueInportName__1__)
  State Estimation_sfcn/2 -> __OutputSSForSFun__/2(__UniqueInportName__2__)
  State Estimation_sfcn/3 -> __OutputSSForSFun__/3(__UniqueInportName__3__)
  State Estimation_sfcn/4 -> __OutputSSForSFun__/4(__UniqueInportName__4__)
  State Estimation_sfcn/5 -> __OutputSSForSFun__/5(__UniqueInportName__5__)
  State Estimation_sfcn/6 -> __OutputSSForSFun__/6(__UniqueInportName__6__)
  State Estimation_sfcn/7 -> __OutputSSForSFun__/7(__UniqueInportName__7__)
  State Estimation_sfcn/8 -> __OutputSSForSFun__/8(__UniqueInportName__8__)
  __OutputSSForSFun__/1("[pn, pe, pd]") -> "[pn, pe, pd]"/1
  __OutputSSForSFun__/2(Va) -> Va/1
  __OutputSSForSFun__/3("[wn, we]") -> "[wn, we]"/1
  __OutputSSForSFun__/4("[Phi, Theta, Psi]") -> "[Phi, Theta, Psi]"/1
  __OutputSSForSFun__/5("[p, q, r]") -> "[p, q, r]"/1
  __OutputSSForSFun__/6(Vg) -> Vg/1
  __OutputSSForSFun__/7(Chi) -> Chi/1
  __OutputSSForSFun__/8(alpha) -> alpha/1

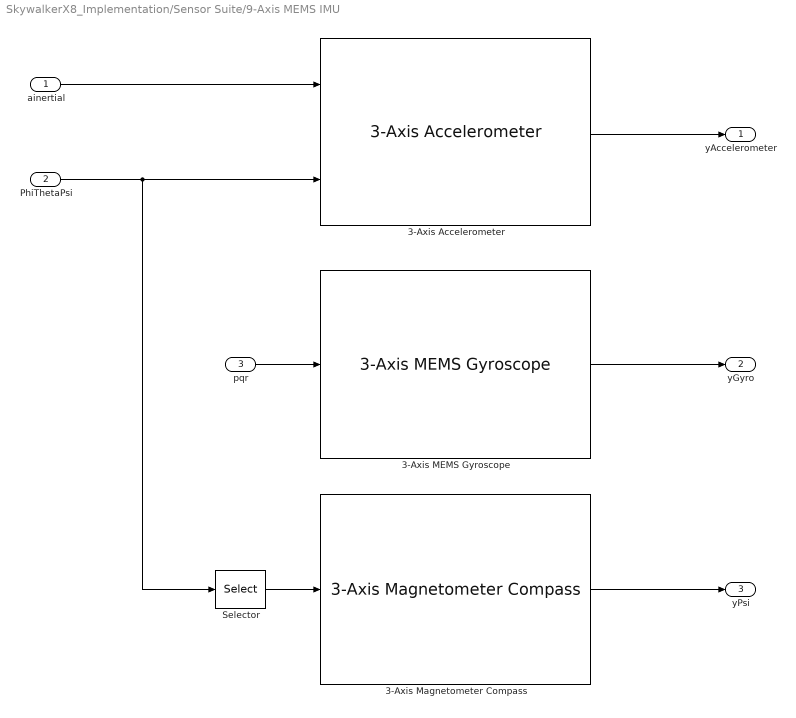
== system SkywalkerX8_Implementation/Sensor Suite/9-Axis MEMS IMU ==
  ainertial : Inport
  PhiThetaPsi : Inport  Port=2
  pqr : Inport  Port=3
  3-Axis Accelerometer : sensors/3-Axis Accelerometer  g=SkywalkerX8.System.Gravity  SampleTime=SkywalkerX8.Sensors.IMU.Accelerometer.SampleTime  accelXNoiseDensity=SkywalkerX8.Sensors.IMU.Accelerometer.X.NoiseDensity  accelYNoiseDensity=SkywalkerX8.Sensors.IMU.Accelerometer.Y.NoiseDensity  accelZNoiseDensity=SkywalkerX8.Sensors.IMU.Accelerometer.Z.NoiseDensity  accelXBandwidthHz=SkywalkerX8.Sensors.IMU.Accelerometer.X.BandwidthHz  accelYBandwidthHz=SkywalkerX8.Sensors.IMU.Accelerometer.Y.BandwidthHz  accelZBandwidthHz=SkywalkerX8.Sensors.IMU.Accelerometer.Z.BandwidthHz  accelXInit=SkywalkerX8.Sensors.IMU.Accelerometer.X.InitialCondition  accelYInit=SkywalkerX8.Sensors.IMU.Accelerometer.Y.InitialCondition  accelZInit=SkywalkerX8.Sensors.IMU.Accelerometer.Z.InitialCondition  accelXUpperSaturation=SkywalkerX8.Sensors.IMU.Accelerometer.X.UpperSat  accelXLowerSaturation=SkywalkerX8.Sensors.IMU.Accelerometer.X.LowerSat  accelYUpperSaturation=SkywalkerX8.Sensors.IMU.Accelerometer.Y.UpperSat  accelYLowerSaturation=SkywalkerX8.Sensors.IMU.Accelerometer.Y.LowerSat  accelZUpperSaturation=SkywalkerX8.Sensors.IMU.Accelerometer.Z.UpperSat  accelZLowerSaturation=SkywalkerX8.Sensors.IMU.Accelerometer.Z.LowerSat  accelXResolution=SkywalkerX8.Sensors.IMU.Accelerometer.X.Resolution  accelYResolution=SkywalkerX8.Sensors.IMU.Accelerometer.Y.Resolution  accelZResolution=SkywalkerX8.Sensors.IMU.Accelerometer.Z.Resolution
  3-Axis MEMS Gyroscope : sensors/3-Axis MEMS Gyroscope  SampleTime=SkywalkerX8.Sensors.IMU.Gyroscope.SampleTime  gyroXNoiseDensity=SkywalkerX8.Sensors.IMU.Gyroscope.X.NoiseDensity  gyroYNoiseDensity=SkywalkerX8.Sensors.IMU.Gyroscope.Y.NoiseDensity  gyroZNoiseDensity=SkywalkerX8.Sensors.IMU.Gyroscope.Z.NoiseDensity  gyroXBandwidthHz=SkywalkerX8.Sensors.IMU.Gyroscope.X.BandwidthHz  gyroYBandwidthHz=SkywalkerX8.Sensors.IMU.Gyroscope.Y.BandwidthHz  gyroZBandwidthHz=SkywalkerX8.Sensors.IMU.Gyroscope.Z.BandwidthHz  gyroXInit=SkywalkerX8.Sensors.IMU.Gyroscope.X.InitialCondition  gyroYInit=SkywalkerX8.Sensors.IMU.Gyroscope.Y.InitialCondition  gyroZInit=SkywalkerX8.Sensors.IMU.Gyroscope.Z.InitialCondition  gyroXUpperSaturation=SkywalkerX8.Sensors.IMU.Gyroscope.X.UpperSat  gyroXLowerSaturation=SkywalkerX8.Sensors.IMU.Gyroscope.X.LowerSat  gyroYUpperSaturation=SkywalkerX8.Sensors.IMU.Gyroscope.Y.UpperSat  gyroYLowerSaturation=SkywalkerX8.Sensors.IMU.Gyroscope.Y.LowerSat  gyroZUpperSaturation=SkywalkerX8.Sensors.IMU.Gyroscope.Z.UpperSat  gyroZLowerSaturation=SkywalkerX8.Sensors.IMU.Gyroscope.Z.LowerSat  gyroXResolution=SkywalkerX8.Sensors.IMU.Gyroscope.X.Resolution  gyroYResolution=SkywalkerX8.Sensors.IMU.Gyroscope.Y.Resolution  gyroZResolution=SkywalkerX8.Sensors.IMU.Gyroscope.Z.Resolution
  3-Axis Magnetometer Compass : sensors/3-Axis Magnetometer Compass  SampleTime=SkywalkerX8.Sensors.IMU.Compass.SampleTime  headingNoiseDensity=SkywalkerX8.Sensors.IMU.Compass.NoiseDensity  headingBandwidthHz=SkywalkerX8.Sensors.IMU.Compass.BandwidthHz  headingInit=SkywalkerX8.Sensors.IMU.Compass.InitialCondition  headingUpperSaturation=SkywalkerX8.Sensors.IMU.Compass.UpperSat  headingLowerSaturation=SkywalkerX8.Sensors.IMU.Compass.LowerSat  headingResolution=SkywalkerX8.Sensors.IMU.Compass.Resolution
  Selector : Selector  InputPortWidth=3  IndexOptions=Index vector (dialog)  Indices=3  OutputSizes=1
  yAccelerometer : Outport
  yGyro : Outport  Port=2
  yPsi : Outport  Port=3
  wires:
  ainertial/1 -> 3-Axis Accelerometer/1
  PhiThetaPsi/1 -> 3-Axis Accelerometer/2, Selector/1
  Selector/1 -> 3-Axis Magnetometer Compass/1
  pqr/1 -> 3-Axis MEMS Gyroscope/1
  3-Axis MEMS Gyroscope/1 -> yGyro/1
  3-Axis Accelerometer/1 -> yAccelerometer/1
  3-Axis Magnetometer Compass/1 -> yPsi/1

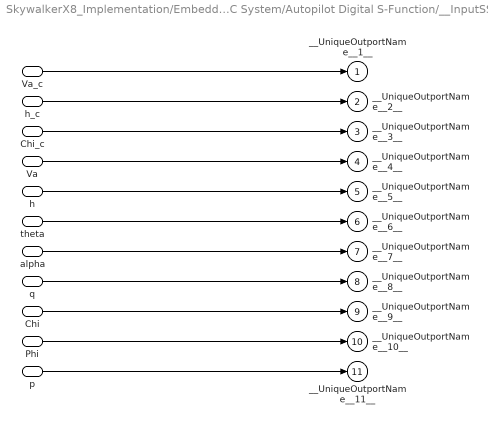
== system SkywalkerX8_Implementation/Embedded GNC System/Autopilot Digital S-Function/__InputSSForSFun__ ==
  Va_c : Inport
  h_c : Inport  Port=2
  Chi_c : Inport  Port=3
  Va : Inport  Port=4
  h : Inport  Port=5
  theta : Inport  Port=6
  alpha : Inport  Port=7
  q : Inport  Port=8
  Chi : Inport  Port=9
  Phi : Inport  Port=10
  p : Inport  Port=11
  __UniqueOutportName__1__ : Outport
  __UniqueOutportName__2__ : Outport  Port=2
  __UniqueOutportName__3__ : Outport  Port=3
  __UniqueOutportName__4__ : Outport  Port=4
  __UniqueOutportName__5__ : Outport  Port=5
  __UniqueOutportName__6__ : Outport  Port=6
  __UniqueOutportName__7__ : Outport  Port=7
  __UniqueOutportName__8__ : Outport  Port=8
  __UniqueOutportName__9__ : Outport  Port=9
  __UniqueOutportName__10__ : Outport  Port=10
  __UniqueOutportName__11__ : Outport  Port=11
  wires:
  Va_c/1 -> __UniqueOutportName__1__/1
  h_c/1 -> __UniqueOutportName__2__/1
  Chi_c/1 -> __UniqueOutportName__3__/1
  Va/1 -> __UniqueOutportName__4__/1
  h/1 -> __UniqueOutportName__5__/1
  theta/1 -> __UniqueOutportName__6__/1
  alpha/1 -> __UniqueOutportName__7__/1
  q/1 -> __UniqueOutportName__8__/1
  Chi/1 -> __UniqueOutportName__9__/1
  Phi/1 -> __UniqueOutportName__10__/1
  p/1 -> __UniqueOutportName__11__/1

== system SkywalkerX8_Implementation/Embedded GNC System/Autopilot Digital S-Function/__OutputSSForSFun__ ==
  __UniqueInportName__1__ : Inport
  __UniqueInportName__2__ : Inport  Port=2
  __UniqueInportName__3__ : Inport  Port=3
  dt : Outport
  der : Outport  Port=2
  del : Outport  Port=3
  wires:
  __UniqueInportName__1__/1 -> dt/1
  __UniqueInportName__2__/1 -> der/1  "der"
  __UniqueInportName__3__/1 -> del/1  "del"

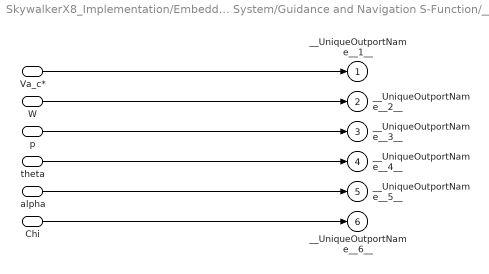
== system SkywalkerX8_Implementation/Embedded GNC System/Guidance and Navigation S-Function/__InputSSForSFun__ ==
  Va_c* : Inport
  W : Inport  Port=2
  p : Inport  Port=3
  theta : Inport  Port=4
  alpha : Inport  Port=5
  Chi : Inport  Port=6
  __UniqueOutportName__1__ : Outport
  __UniqueOutportName__2__ : Outport  Port=2
  __UniqueOutportName__3__ : Outport  Port=3
  __UniqueOutportName__4__ : Outport  Port=4
  __UniqueOutportName__5__ : Outport  Port=5
  __UniqueOutportName__6__ : Outport  Port=6
  wires:
  Va_c*/1 -> __UniqueOutportName__1__/1
  W/1 -> __UniqueOutportName__2__/1
  p/1 -> __UniqueOutportName__3__/1
  theta/1 -> __UniqueOutportName__4__/1
  alpha/1 -> __UniqueOutportName__5__/1
  Chi/1 -> __UniqueOutportName__6__/1

== system SkywalkerX8_Implementation/Embedded GNC System/Guidance and Navigation S-Function/__OutputSSForSFun__ ==
  __UniqueInportName__1__ : Inport
  __UniqueInportName__2__ : Inport  Port=2
  __UniqueInportName__3__ : Inport  Port=3
  Va_c : Outport
  h_c : Outport  Port=2
  Chi_c : Outport  Port=3
  wires:
  __UniqueInportName__1__/1 -> Va_c/1  "Va_c"
  __UniqueInportName__2__/1 -> h_c/1  "h_c"
  __UniqueInportName__3__/1 -> Chi_c/1  "Chi_c"

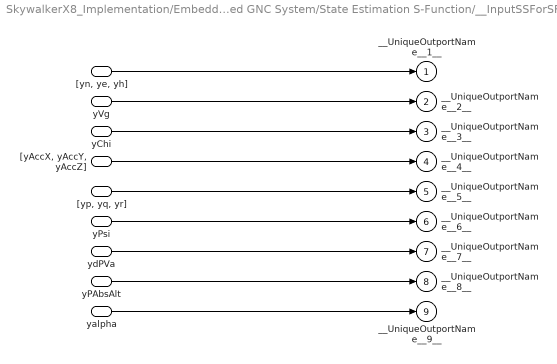
== system SkywalkerX8_Implementation/Embedded GNC System/State Estimation S-Function/__InputSSForSFun__ ==
  "[yn, ye, yh]" : Inport  PortDimensions=3
  yVg : Inport  Port=2
  yChi : Inport  Port=3
  "[yAccX, yAccY, yAccZ]" : Inport  Port=4  PortDimensions=3
  "[yp, yq, yr]" : Inport  Port=5  PortDimensions=3
  yPsi : Inport  Port=6
  ydPVa : Inport  Port=7
  yPAbsAlt : Inport  Port=8
  yalpha : Inport  Port=9
  __UniqueOutportName__1__ : Outport
  __UniqueOutportName__2__ : Outport  Port=2
  __UniqueOutportName__3__ : Outport  Port=3
  __UniqueOutportName__4__ : Outport  Port=4
  __UniqueOutportName__5__ : Outport  Port=5
  __UniqueOutportName__6__ : Outport  Port=6
  __UniqueOutportName__7__ : Outport  Port=7
  __UniqueOutportName__8__ : Outport  Port=8
  __UniqueOutportName__9__ : Outport  Port=9
  wires:
  "[yn, ye, yh]"/1 -> __UniqueOutportName__1__/1
  yVg/1 -> __UniqueOutportName__2__/1
  yChi/1 -> __UniqueOutportName__3__/1
  "[yAccX, yAccY, yAccZ]"/1 -> __UniqueOutportName__4__/1
  "[yp, yq, yr]"/1 -> __UniqueOutportName__5__/1
  yPsi/1 -> __UniqueOutportName__6__/1
  ydPVa/1 -> __UniqueOutportName__7__/1
  yPAbsAlt/1 -> __UniqueOutportName__8__/1
  yalpha/1 -> __UniqueOutportName__9__/1

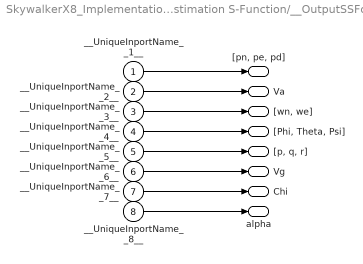
== system SkywalkerX8_Implementation/Embedded GNC System/State Estimation S-Function/__OutputSSForSFun__ ==
  __UniqueInportName__1__ : Inport
  __UniqueInportName__2__ : Inport  Port=2
  __UniqueInportName__3__ : Inport  Port=3
  __UniqueInportName__4__ : Inport  Port=4
  __UniqueInportName__5__ : Inport  Port=5
  __UniqueInportName__6__ : Inport  Port=6
  __UniqueInportName__7__ : Inport  Port=7
  __UniqueInportName__8__ : Inport  Port=8
  "[pn, pe, pd]" : Outport
  Va : Outport  Port=2
  "[wn, we]" : Outport  Port=3
  "[Phi, Theta, Psi]" : Outport  Port=4
  "[p, q, r]" : Outport  Port=5
  Vg : Outport  Port=6
  Chi : Outport  Port=7
  alpha : Outport  Port=8
  wires:
  __UniqueInportName__1__/1 -> "[pn, pe, pd]"/1
  __UniqueInportName__2__/1 -> Va/1
  __UniqueInportName__3__/1 -> "[wn, we]"/1
  __UniqueInportName__4__/1 -> "[Phi, Theta, Psi]"/1
  __UniqueInportName__5__/1 -> "[p, q, r]"/1
  __UniqueInportName__6__/1 -> Vg/1
  __UniqueInportName__7__/1 -> Chi/1
  __UniqueInportName__8__/1 -> alpha/1

== matlab function SkywalkerX8_Implementation/SkywalkerX8 Aircraft + Aerodynamics Observable Feedback/Rotatation Body to Vehicle ==
  data: PhiThetaPsi input; wnwewd output; uwvwww input
function wnwewd = fcn(PhiThetaPsi, uwvwww)

    Phi = PhiThetaPsi(1);
    Theta = PhiThetaPsi(2);
    Psi = PhiThetaPsi(3);

    Rvb = [cos(Theta)*cos(Psi)                             , cos(Theta)*sin(Psi)                             , -sin(Theta)        ;
           sin(Phi)*sin(Theta)*cos(Psi) - cos(Phi)*sin(Psi), sin(Phi)*sin(Theta)*sin(Psi) + cos(Phi)*cos(Psi), sin(Phi)*cos(Theta);
           cos(Phi)*sin(Theta)*cos(Psi) + sin(Phi)*sin(Psi), cos(Phi)*sin(Theta)*sin(Psi) - sin(Phi)*cos(Psi), cos(Phi)*cos(Theta)];

    uwvwww = reshape(uwvwww, 3, 1);

    wnwewd = Rvb\uwvwww;
    
end

== matlab function SkywalkerX8_Implementation/SkywalkerX8 Aircraft + Aerodynamics Observable Feedback/Rotatation Vehicle to Body ==
  data: PhiThetaPsi input; uwvwww output; wnwewd input
function uwvwww = fcn(PhiThetaPsi, wnwewd)

    Phi = PhiThetaPsi(1);
    Theta = PhiThetaPsi(2);
    Psi = PhiThetaPsi(3);

    Rvb = [cos(Theta)*cos(Psi)                             , cos(Theta)*sin(Psi)                             , -sin(Theta)        ;
           sin(Phi)*sin(Theta)*cos(Psi) - cos(Phi)*sin(Psi), sin(Phi)*sin(Theta)*sin(Psi) + cos(Phi)*cos(Psi), sin(Phi)*cos(Theta);
           cos(Phi)*sin(Theta)*cos(Psi) + sin(Phi)*sin(Psi), cos(Phi)*sin(Theta)*sin(Psi) - sin(Phi)*cos(Psi), cos(Phi)*cos(Theta)];

    wnwewed = reshape(wnwewd, 3, 1);

    uwvwww = Rvb*wnwewed;
    
end
